simulink model "REGX_LINEARIZOVANE_simulink"  (R2019b)
settings: Solver=FixedStepAuto  StartTime=0.0  StopTime=5  FixedStep=0.01  MaxStep=0.01  RelTol=1e-3
undefined symbols (not defined in the file or in its folder): Arx, Brx, Crx, Krx, x0rx, x1k_rx
settings Model: Creator=jakub  LastModifiedBy=z004506p

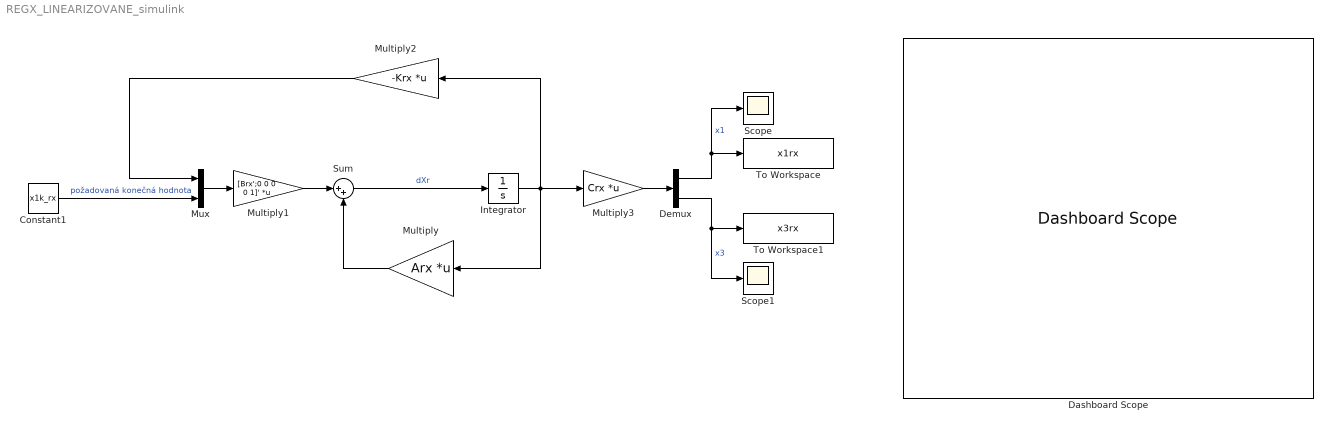
== system REGX_LINEARIZOVANE_simulink ==
  Constant1 : Constant  Value=x1k_rx
  Dashboard Scope : DashboardScope  Ymin=-1  Ymax=1
  Demux : Demux  Outputs=2
  Integrator : Integrator  InitialCondition=x0rx
  Multiply : Gain  Gain=Arx  Multiplication=Matrix(K*u) (u vector)
  Multiply1 : Gain  Gain=[Brx';0 0 0 0 1]'  Multiplication=Matrix(K*u) (u vector)
  Multiply2 : Gain  Gain=-Krx  Multiplication=Matrix(K*u) (u vector)
  Multiply3 : Gain  Gain=Crx  Multiplication=Matrix(K*u) (u vector)
  Mux : Mux  Inputs=2
  Scope : Scope
  Scope1 : Scope
  Sum : Sum  Inputs=|++
  To Workspace : ToWorkspace  VariableName=x1rx  SaveFormat=Timeseries  SampleTime=-1
  To Workspace1 : ToWorkspace  VariableName=x3rx  SaveFormat=Timeseries  SampleTime=-1
  wires:
  Sum/1 -> Integrator/1  "dXr"
  Multiply1/1 -> Sum/1
  Multiply/1 -> Sum/2
  Multiply2/1 -> Mux/1
  Multiply3/1 -> Demux/1
  Demux/1 -> To Workspace/1, Scope/1  "x1"
  Demux/2 -> To Workspace1/1, Scope1/1  "x3"
  Constant1/1 -> Mux/2  "požadovaná konečná hodnota"
  Mux/1 -> Multiply1/1
  Integrator/1 -> Multiply/1, Multiply2/1, Multiply3/1
